simulink model "plant"  (R2023a)
settings: Solver=VariableStepAuto  StartTime=0.0  StopTime=TF  RelTol=1e-3
values from neighbouring files (symbols this model uses):
  x0 = [85; 0; 0; 0; 0; 0; 0; 0.1; 0; 44.94028*pi/180; -73.09747*pi/180; 3000*0.2808]    [init.m]
undefined symbols (not defined in the file or in its folder): aircraft_6DOF_model
libraries: aerolibfltsims x2, aerolibanimutils x1
settings Model: Creator=Hegde  LastModifiedBy=Hegde

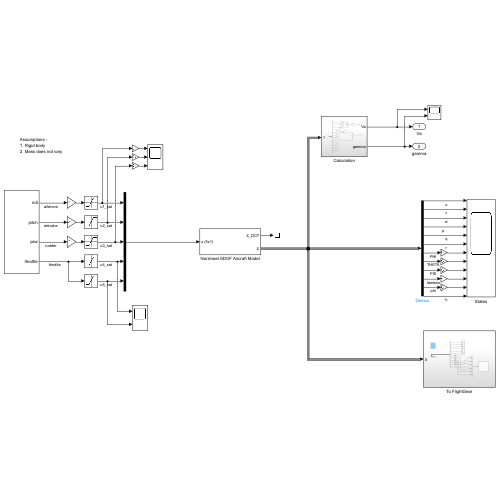
[thumbnail: Simulink's stored preview of the top-level diagram]
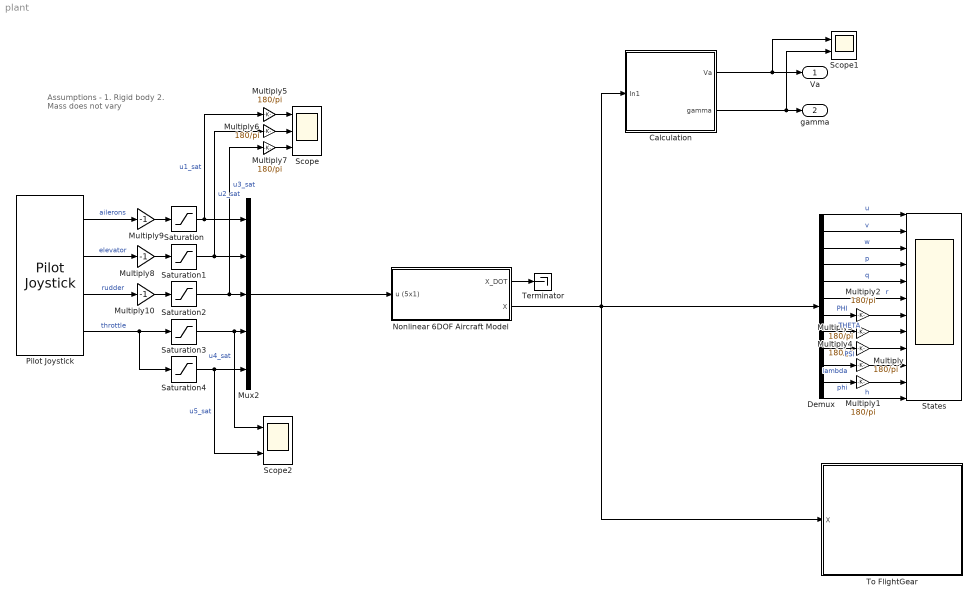
== system plant ==
  note: Assumptions -
      | 1. Rigid body
      | 2. Mass does not vary
  Calculation : Subsystem
  Demux : Demux  Outputs=12
  Multiply{,1..7} (8 alike) : Gain  Gain=180/pi
  Multiply10 : Gain  Gain=-1
  Multiply8 : Gain  Gain=-1
  Multiply9 : Gain  Gain=-1
  Mux2 : Mux  Inputs=5
  Nonlinear 6DOF Aircraft Model : Subsystem
  Pilot Joystick : aerolibanimutils/Pilot Joystick  JoystickID=Joystick1  OutputConfiguration=FourAxis  SampleTime=1/30
  Saturation : Saturate  UpperLimit=25 * pi/180  LowerLimit=-25 * pi/180
  Saturation1 : Saturate  UpperLimit=10 * pi/180  LowerLimit=-25 * pi/180
  Saturation2 : Saturate  UpperLimit=30 * pi/180  LowerLimit=-30 * pi/180
  Saturation3 : Saturate  UpperLimit=1  LowerLimit=0
  Saturation4 : Saturate  UpperLimit=1  LowerLimit=0
  Scope : Scope  NumInputPorts=3
  Scope1 : Scope  NumInputPorts=2
  Scope2 : Scope  NumInputPorts=2
  States : Scope  NumInputPorts=12
  Terminator : Terminator
  To FlightGear : Subsystem
  Va : Outport
  gamma : Outport  Port=2
  wires:
  Demux/1 -> States/1  "u"
  Demux/2 -> States/2  "v"
  Demux/3 -> States/3  "w"
  Demux/4 -> States/4  "p"
  Demux/5 -> States/5  "q"
  Demux/6 -> States/6  "r"
  Demux/7 -> Multiply2/1  "PHI"
  Demux/8 -> Multiply3/1  "THETA"
  Demux/9 -> Multiply4/1  "PSI"
  Calculation/2(gamma) -> gamma/1, Scope1/2
  Calculation/1(Va) -> Va/1, Scope1/1
  Mux2/1 -> Nonlinear 6DOF Aircraft Model/1(u (5x1))
  Pilot Joystick/1 -> Multiply9/1  "ailerons"
  Pilot Joystick/2 -> Multiply8/1  "elevator"
  Pilot Joystick/3 -> Multiply10/1  "rudder"
  Pilot Joystick/4 -> Saturation3/1, Saturation4/1  "throttle"
  Demux/10 -> Multiply/1  "lambda"
  Demux/11 -> Multiply1/1  "phi"
  Demux/12 -> States/12  "h"
  Multiply/1 -> States/10
  Multiply1/1 -> States/11
  Multiply2/1 -> States/7
  Multiply3/1 -> States/8
  Multiply4/1 -> States/9
  Nonlinear 6DOF Aircraft Model/2(X) -> Calculation/1(In1), Demux/1, To FlightGear/1(X)
  Saturation/1 -> Mux2/1, Multiply5/1  "u1_sat"
  Saturation1/1 -> Multiply6/1, Mux2/2  "u2_sat"
  Saturation2/1 -> Multiply7/1, Mux2/3  "u3_sat"
  Saturation3/1 -> Scope2/1, Mux2/4  "u4_sat"
  Saturation4/1 -> Mux2/5, Scope2/2  "u5_sat"
  Multiply5/1 -> Scope/1
  Multiply6/1 -> Scope/2
  Multiply7/1 -> Scope/3
  Multiply8/1 -> Saturation1/1
  Multiply9/1 -> Saturation/1
  Multiply10/1 -> Saturation2/1
  Nonlinear 6DOF Aircraft Model/1(X_DOT) -> Terminator/1

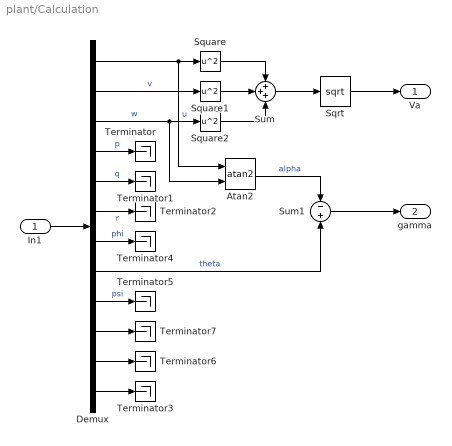
== system plant/Calculation ==
  In1 : Inport
  Atan2 : Trigonometry  Operator=atan2
  Demux : Demux  Outputs=12
  Sqrt : Sqrt
  Square : Math  Operator=square
  Square1 : Math  Operator=square
  Square2 : Math  Operator=square
  Sum : Sum  Inputs=+++
  Sum1 : Sum  Inputs=-+
  Terminator{,1..7} (8 alike) : Terminator
  Va : Outport
  gamma : Outport  Port=2
  wires:
  Demux/1 -> Atan2/1, Square/1  "u"
  Square/1 -> Sum/1
  Demux/9 -> Terminator5/1  "psi"
  Demux/5 -> Terminator1/1  "q"
  Demux/3 -> Square2/1, Atan2/2  "w"
  In1/1 -> Demux/1
  Demux/2 -> Square1/1  "v"
  Demux/6 -> Terminator2/1  "r"
  Atan2/1 -> Sum1/1  "alpha"
  Demux/4 -> Terminator/1  "p"
  Sum1/1 -> gamma/1
  Square2/1 -> Sum/3
  Sum/1 -> Sqrt/1
  Demux/7 -> Terminator4/1  "phi"
  Demux/8 -> Sum1/2  "theta"
  Square1/1 -> Sum/2
  Sqrt/1 -> Va/1
  Demux/12 -> Terminator3/1
  Demux/10 -> Terminator7/1
  Demux/11 -> Terminator6/1

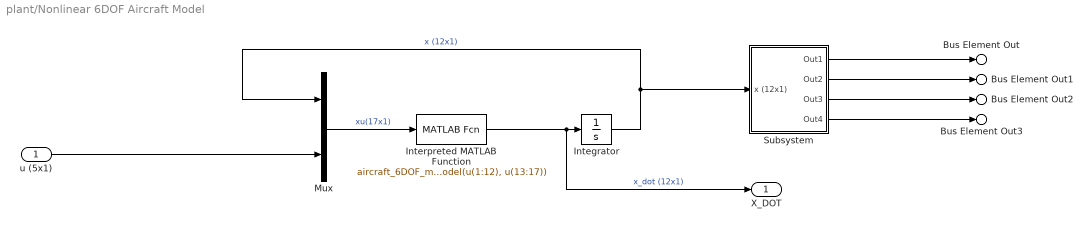
== system plant/Nonlinear 6DOF Aircraft Model ==
  u (5x1) : Inport
  Integrator : Integrator  InitialCondition=x0
  Interpreted MATLAB Function : MATLABFcn  MATLABFcn=aircraft_6DOF_model(u(1:12), u(13:17))
  Mux : Mux  Inputs=2
  Subsystem : Subsystem
  X_DOT : Outport
  Bus Element Out : Outport  Port=2  PortName=X  Element=VEL_K_G_B_E
  Bus Element Out1 : Outport  Port=2  PortName=X  Element=OMEGA_K_OB_B_B
  Bus Element Out2 : Outport  Port=2  PortName=X  Element=ATT
  Bus Element Out3 : Outport  Port=2  PortName=X  Element=POS_WSG-84
  wires:
  Integrator/1 -> Subsystem/1(x (12x1)), Mux/1  "x (12x1)"
  Interpreted MATLAB Function/1 -> X_DOT/1, Integrator/1  "x_dot (12x1)"
  Mux/1 -> Interpreted MATLAB Function/1  "xu(17x1)"
  u (5x1)/1 -> Mux/2
  Subsystem/1(Out1) -> Bus Element Out/1
  Subsystem/2(Out2) -> Bus Element Out1/1
  Subsystem/3(Out3) -> Bus Element Out2/1
  Subsystem/4(Out4) -> Bus Element Out3/1

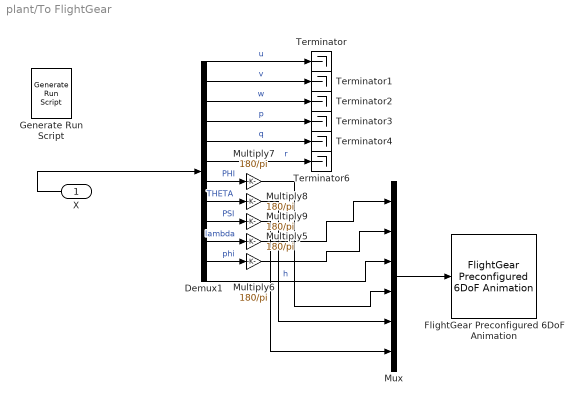
== system plant/To FlightGear ==
  X : Inport
  Demux1 : Demux  Outputs=12
  FlightGear Preconfigured 6DoF Animation : aerolibfltsims/FlightGear Preconfigured 6DoF Animation  xFlightGearVersion=v2019.1  DestinationIpAddress=127.0.0.1  DestinationPort=5502  SampleTime=1/30  packetVersion=24
  Generate Run Script : aerolibfltsims/Generate Run Script  Architecture=Default  dataFlow=Send  GeometryModelName=c172p  AirportId=KSFO  RunwayId=10L  InitialAltitude=3000*0.2808  InitialHeading=113  OffsetDistance=4.72  OffsetAzimuth=0  InstallScenery=on  DisableShaders=on  OriginAddress=127.0.0.1  DestinationPort=5502  OriginPort=5505  LocalAddress=127.0.0.1  OutputFileName=runfg.bat  FlightGearBaseDirectory=C:\Program Files\FlightGear 2024.1
  Multiply{5..9} (5 alike) : Gain  Gain=180/pi
  Mux : Mux  Inputs=6
  Terminator{,1..4,6} (6 alike) : Terminator
  wires:
  Demux1/4 -> Terminator3/1  "p"
  Demux1/10 -> Multiply5/1  "lambda"
  Demux1/7 -> Multiply7/1  "PHI"
  Multiply7/1 -> Mux/4
  Demux1/1 -> Terminator/1  "u"
  Demux1/11 -> Multiply6/1  "phi"
  Demux1/12 -> Mux/3  "h"
  Demux1/9 -> Multiply9/1  "PSI"
  Demux1/8 -> Multiply8/1  "THETA"
  Multiply5/1 -> Mux/1
  Mux/1 -> FlightGear Preconfigured 6DoF Animation/1
  Multiply9/1 -> Mux/6
  Demux1/6 -> Terminator6/1  "r"
  Multiply8/1 -> Mux/5
  Demux1/3 -> Terminator2/1  "w"
  Demux1/2 -> Terminator1/1  "v"
  Multiply6/1 -> Mux/2
  Demux1/5 -> Terminator4/1  "q"
  X/1 -> Demux1/1

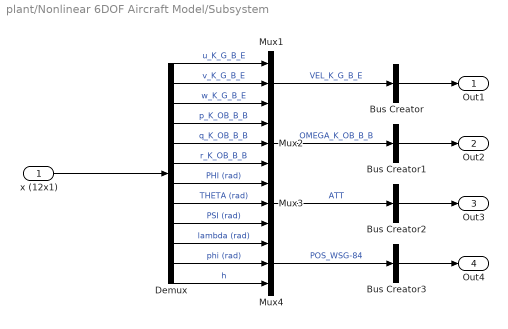
== system plant/Nonlinear 6DOF Aircraft Model/Subsystem ==
  x (12x1) : Inport
  Bus Creator{,1..3} (4 alike) : BusCreator  Inputs=1
  Demux : Demux  Outputs=12
  Mux{1..4} (4 alike) : Mux  Inputs=3
  Out1 : Outport
  Out2 : Outport  Port=2
  Out3 : Outport  Port=3
  Out4 : Outport  Port=4
  wires:
  Demux/8 -> Mux3/2  "THETA (rad)"
  Demux/10 -> Mux4/1  "lambda (rad)"
  Demux/9 -> Mux3/3  "PSI (rad)"
  Demux/1 -> Mux1/1  "u_K_G_B_E"
  Demux/12 -> Mux4/3  "h"
  Demux/4 -> Mux2/1  "p_K_OB_B_B"
  Demux/6 -> Mux2/3  "r_K_OB_B_B"
  Demux/2 -> Mux1/2  "v_K_G_B_E"
  Demux/5 -> Mux2/2  "q_K_OB_B_B"
  Demux/11 -> Mux4/2  "phi (rad)"
  Mux1/1 -> Bus Creator/1  "VEL_K_G_B_E"
  Demux/3 -> Mux1/3  "w_K_G_B_E"
  Bus Creator1/1 -> Out2/1
  Demux/7 -> Mux3/1  "PHI (rad)"
  Bus Creator3/1 -> Out4/1
  Mux3/1 -> Bus Creator2/1  "ATT"
  Bus Creator/1 -> Out1/1
  Mux4/1 -> Bus Creator3/1  "POS_WSG-84"
  Mux2/1 -> Bus Creator1/1  "OMEGA_K_OB_B_B"
  Bus Creator2/1 -> Out3/1
  x (12x1)/1 -> Demux/1
